simulink library "Library_SII_2018"  (R2018b)
settings: Solver=ode45  StartTime=0.0  StopTime=10.0  RelTol=1e-3  EnableMultiTasking=on
undefined symbols (not defined in the file or in its folder): coder, gcbh, r, simscape
libraries: fl_lib x157, nesl_utility x81, Library_SII2 x44, simulink x17, powerlib x12, mblibv1 x11, Simscape_SII_lib x11, elec_lib x10, Pneumatic_lib x4, $bdroot x2, peRmsMeasurement x1, powerlib_extras x1
(part 6 of 6)

== system Library_SII_2018/Thermique/Paroi (avec convection) ==
  Capacité : fl_lib/Thermal/Thermal Elements/Thermal Mass  mass=masse kg  sp_heat=c J/kg/K  T_specify=on  T_priority=High  T=Ti K  T_nominal_specify=off  T_nominal_unit=K  T_nominal_value=1  Q_specify=off  Q_priority=High  Q=0 J/s  Q_nominal_specify=off  Q_nominal_unit=W  Q_nominal_value=1
  Conduction ext : fl_lib/Thermal/Thermal Elements/Conductive Heat Transfer  area=s m^2  thickness=e/2 cm  th_cond=lambda W/(m*K)  T_specify=off  T_priority=High  T=0 K  T_nominal_specify=off  T_nominal_unit=K  T_nominal_value=1  Q_specify=off  Q_priority=High  Q=0 J/s  Q_nominal_specify=off  Q_nominal_unit=W  Q_nominal_value=1
      settings: SourceProductName=Simscape
  Conduction int : fl_lib/Thermal/Thermal Elements/Conductive Heat Transfer  area=s m^2  thickness=e/2 cm  th_cond=lambda W/(m*K)  T_specify=off  T_priority=High  T=0 K  T_nominal_specify=off  T_nominal_unit=K  T_nominal_value=1  Q_specify=off  Q_priority=High  Q=0 J/s  Q_nominal_specify=off  Q_nominal_unit=W  Q_nominal_value=1
      settings: SourceProductName=Simscape
  Ideal Heat Flow Sensor. : fl_lib/Thermal/Thermal Sensors/Heat Flow Rate Sensor
      settings: SourceProductName=Simscape  SourceProductBaseCode=SS
  Ideal Heat Flow Sensor.1 : fl_lib/Thermal/Thermal Sensors/Heat Flow Rate Sensor
      settings: SourceProductName=Simscape  SourceProductBaseCode=SS
  Ideal Temperature Sensor : fl_lib/Thermal/Thermal Sensors/Temperature Sensor
  PS-Simulink Converter : nesl_utility/PS-Simulink Converter  PhysicalDomain=network_engine_domain  SubClassName=ps_output  LeftPortType=input  RightPortType=output  PseudoPeriodic=off  Frequencies=[]  Unit=degC  AffineConversion=on
  PS2S : nesl_utility/PS-Simulink Converter  PhysicalDomain=network_engine_domain  SubClassName=ps_output  LeftPortType=input  RightPortType=output  PseudoPeriodic=off  Frequencies=[]  Unit=J/s  AffineConversion=off
  PS2S1 : nesl_utility/PS-Simulink Converter  PhysicalDomain=network_engine_domain  SubClassName=ps_output  LeftPortType=input  RightPortType=output  PseudoPeriodic=off  Frequencies=[]  Unit=J/s  AffineConversion=off
  Thermal Reference : fl_lib/Thermal/Thermal Elements/Thermal Reference
  Int : PMIOPort  Side=Left
  Ext : PMIOPort  Port=2  Side=Right
  Ray : PMIOPort  Port=3  Side=Right
  T : Outport
  Fext : Outport  Port=2
  Fint : Outport  Port=3
  wires:
  PS2S1/1 -> Fint/1
  PS2S/1 -> Fext/1
  PS-Simulink Converter/1 -> T/1
  connections:
  Conduction int/RConn1 -- Ideal Heat Flow Sensor.1/LConn1
  Ideal Heat Flow Sensor.1/RConn1 -- PS2S1/LConn1
  Ideal Heat Flow Sensor./RConn1 -- PS2S/LConn1
  Conduction ext/LConn1 -- Ideal Heat Flow Sensor./RConn2
  Conduction ext/RConn1 -- Ext/RConn1
  Int/RConn1 -- Conduction int/LConn1
  Ideal Heat Flow Sensor./LConn1 -- Ideal Temperature Sensor/LConn1 -- Ray/RConn1 -- Ideal Heat Flow Sensor.1/RConn2 -- Capacité/LConn1
  PS-Simulink Converter/LConn1 -- Ideal Temperature Sensor/RConn2
  Thermal Reference/LConn1 -- Ideal Temperature Sensor/RConn1

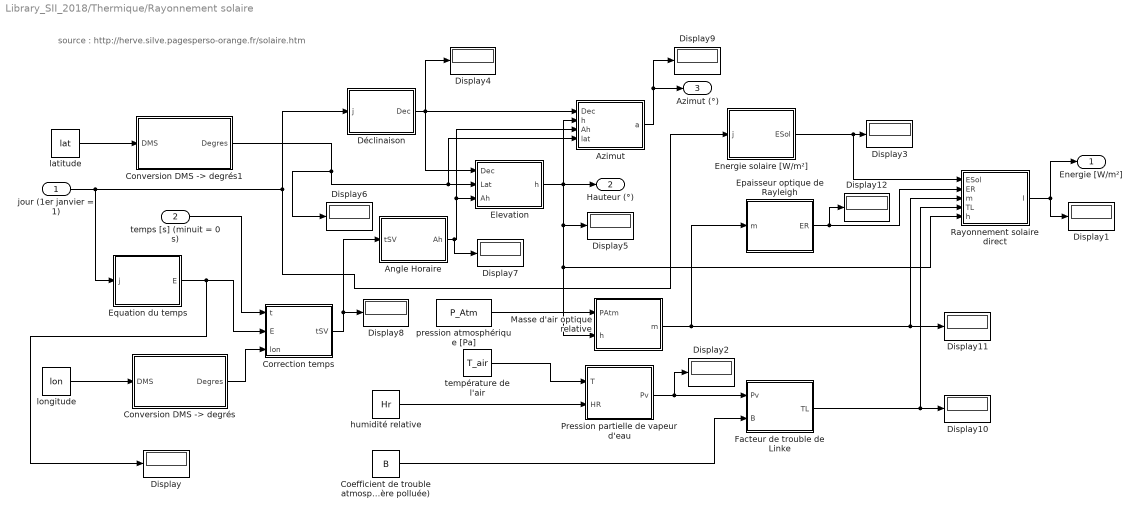
== system Library_SII_2018/Thermique/Rayonnement solaire ==
  note: source : http://herve.silve.pagesperso-orange.fr/solaire.htm
  jour (1er janvier = 1) : Inport
  temps [s] (minuit = 0 s) : Inport  Port=2
  Angle Horaire : MATLAB Function  TreatAsAtomicUnit=on
  Azimut : MATLAB Function  TreatAsAtomicUnit=on
  Coefficient de trouble atmosphérique B = 0,02 pour un lieu situé en montagne B = 0,05 pour un lieu rural B = 0,10 pour un lieu urbain B = 0,20 pour un lieu industriel (atmosphère polluée) : Constant  Value=B
  "Conversion DMS -> degrés" : MATLAB Function  TreatAsAtomicUnit=on
  "Conversion DMS -> degrés1" : MATLAB Function  TreatAsAtomicUnit=on
  Correction temps : MATLAB Function  TreatAsAtomicUnit=on
  Display{,1..12} (13 alike) : Display
  Déclinaison : MATLAB Function  TreatAsAtomicUnit=on
  Elevation : MATLAB Function  TreatAsAtomicUnit=on
  Energie solaire [W/m²] : MATLAB Function  TreatAsAtomicUnit=on
  Epaisseur optique de Rayleigh : MATLAB Function  TreatAsAtomicUnit=on
  Equation du temps : MATLAB Function  TreatAsAtomicUnit=on
  Facteur de trouble de Linke : MATLAB Function  TreatAsAtomicUnit=on
  Masse d'air optique relative : MATLAB Function  TreatAsAtomicUnit=on
  Pression partielle de vapeur d'eau : MATLAB Function  TreatAsAtomicUnit=on
  Rayonnement solaire direct : MATLAB Function  TreatAsAtomicUnit=on
  humidité relative : Constant  Value=Hr
  latitude : Constant  Value=lat
  longitude : Constant  Value=lon
  pression atmosphérique [Pa] : Constant  Value=P_Atm
  température de l'air : Constant  Value=T_air
  Energie [W/m²] : Outport
  Hauteur (°) : Outport  Port=2
  Azimut (°) : Outport  Port=3
  wires:
  Epaisseur optique de Rayleigh/1(ER) -> Display12/1, Rayonnement solaire direct/2(ER)
  Energie solaire [W/m²]/1(ESol) -> Display3/1, Rayonnement solaire direct/1(ESol)
  humidité relative/1 -> Pression partielle de vapeur d'eau/2(HR)
  Rayonnement solaire direct/1(I) -> Energie [W/m²]/1, Display1/1
  température de l'air/1 -> Pression partielle de vapeur d'eau/1(T)
  jour (1er janvier = 1)/1 -> Equation du temps/1(j), Déclinaison/1(j), Energie solaire [W/m²]/1(j)
  Masse d'air optique relative/1(m) -> Display11/1, Rayonnement solaire direct/3(m), Epaisseur optique de Rayleigh/1(m)
  Equation du temps/1(E) -> Display/1, Correction temps/2(E)
  pression atmosphérique [Pa]/1 -> Masse d'air optique relative/1(PAtm)
  Elevation/1(h) -> Azimut/2(h), Masse d'air optique relative/2(h), Rayonnement solaire direct/5(h), Display5/1, Hauteur (°)/1
  Pression partielle de vapeur d'eau/1(Pv) -> Facteur de trouble de Linke/1(Pv), Display2/1
  Facteur de trouble de Linke/1(TL) -> Rayonnement solaire direct/4(TL), Display10/1
  Déclinaison/1(Dec) -> Display4/1, Azimut/1(Dec), Elevation/1(Dec)
  temps [s] (minuit = 0 s)/1 -> Correction temps/1(t)
  Angle Horaire/1(Ah) -> Display7/1, Azimut/3(Ah), Elevation/3(Ah)
  Coefficient de trouble atmosphérique B = 0,02 pour un lieu situé en montagne B = 0,05 pour un lieu rural B = 0,10 pour un lieu urbain B = 0,20 pour un lieu industriel (atmosphère polluée)/1 -> Facteur de trouble de Linke/2(B)
  Correction temps/1(tSV) -> Display8/1, Angle Horaire/1(tSV)
  longitude/1 -> "Conversion DMS -> degrés"/1(DMS)
  "Conversion DMS -> degrés"/1(Degres) -> Correction temps/3(lon)
  "Conversion DMS -> degrés1"/1(Degres) -> Display6/1, Elevation/2(Lat), Azimut/4(lat)
  latitude/1 -> "Conversion DMS -> degrés1"/1(DMS)
  Azimut/1(a) -> Azimut (°)/1, Display9/1

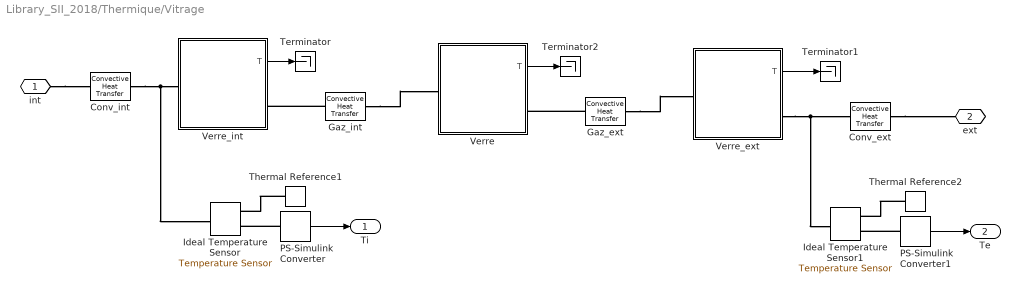
== system Library_SII_2018/Thermique/Vitrage ==
  Conv_ext : fl_lib/Thermal/Thermal Elements/Convective Heat Transfer  area=s m^2  heat_tr_coeff=23 W/(m^2 * K)  T_specify=off  T_priority=High  T=0 K  T_nominal_specify=off  T_nominal_unit=K  T_nominal_value=1  Q_specify=off  Q_priority=High  Q=0 J/s  Q_nominal_specify=off  Q_nominal_unit=W  Q_nominal_value=1
  Conv_int : fl_lib/Thermal/Thermal Elements/Convective Heat Transfer  area=s m^2  heat_tr_coeff=8 W/(m^2 * K)  T_specify=off  T_priority=High  T=0 K  T_nominal_specify=off  T_nominal_unit=K  T_nominal_value=1  Q_specify=off  Q_priority=High  Q=0 J/s  Q_nominal_specify=off  Q_nominal_unit=W  Q_nominal_value=1
  Gaz_ext : fl_lib/Thermal/Thermal Elements/Convective Heat Transfer  area=s m^2  heat_tr_coeff=1e12 W/(m^2 * K)  T_specify=off  T_priority=High  T=0 K  T_nominal_specify=off  T_nominal_unit=K  T_nominal_value=1  Q_specify=off  Q_priority=High  Q=0 J/s  Q_nominal_specify=off  Q_nominal_unit=W  Q_nominal_value=1
  Gaz_int : fl_lib/Thermal/Thermal Elements/Convective Heat Transfer  area=s m^2  heat_tr_coeff=1e12 W/(m^2 * K)  T_specify=off  T_priority=High  T=0 K  T_nominal_specify=off  T_nominal_unit=K  T_nominal_value=1  Q_specify=off  Q_priority=High  Q=0 J/s  Q_nominal_specify=off  Q_nominal_unit=W  Q_nominal_value=1
  Ideal Temperature Sensor : fl_lib/Thermal/Thermal Sensors/Temperature Sensor
  Ideal Temperature Sensor1 : fl_lib/Thermal/Thermal Sensors/Temperature Sensor
  PS-Simulink Converter : nesl_utility/PS-Simulink Converter  PhysicalDomain=network_engine_domain  SubClassName=ps_output  LeftPortType=input  RightPortType=output  PseudoPeriodic=off  Frequencies=[]  Unit=degC  AffineConversion=on
  PS-Simulink Converter1 : nesl_utility/PS-Simulink Converter  PhysicalDomain=network_engine_domain  SubClassName=ps_output  LeftPortType=input  RightPortType=output  PseudoPeriodic=off  Frequencies=[]  Unit=degC  AffineConversion=on
  Terminator : Terminator
  Terminator1 : Terminator
  Terminator2 : Terminator
  Thermal Reference1 : fl_lib/Thermal/Thermal Elements/Thermal Reference
  Thermal Reference2 : fl_lib/Thermal/Thermal Elements/Thermal Reference
  Verre : Subsystem  mask(Paroi){m=Verre, d=off, lambda=1e12, c=720, mv=2530, s=s, e=6, Ti=Ti}
      mask prompts: m "Matériau"; d "Utiliser des valeurs personnalisées"; lambda "Conductivité thermique (W.m<sup>-1</sup>.K<sup>-1</sup>)"; c "Capacité thermique (J.kg<sup>-1</sup>.K<sup>-1</sup>)"; mv "Masse volumique (kg/m<sup>3</sup>)"; s "Surface de la paroi (m<sup>2</sup>)"; e "Epaisseur de la paroi (cm)"; Ti "Température initiale (°C)"
      mask help:
      | Modèle d'une paroi opaque (transmission de la chaleur par conduction).
      |
      | 1) Choisir un matériau
      | ou bien indiquer les caractéristiques thermiques d'un matériau
      | - Conductivité thermique (W.m-1.K-1)
      | - Capacité thermique (J.kg-1.K-1)
      | - Masse volumique (kg/m3)
      |
      | 2) Indiquer les dimensions de la paroi :
      | - Surface (m²)
      | - Epaisseur (cm)
      |
      | 3) Préciser la température initiale (°C)
      |
      | ==> Sortie :
      | T = Température au coeur de la paroi (°C)
      mask init:
      | % Conversion de la température
      | Ti = 273.15+Ti;
      | 
      | % Calcul de la masse
      | masse = mv * s * e / 100;
      | 
      | CaractMateriaux;
      mask Help:
      | Modèle d'une paroi opaque (transmission de la chaleur par conduction).
      | 
      | 1) Choisir un matériau
      | ou bien indiquer les caractéristiques thermiques d'un matériau
      | - Conductivité thermique (W.m<sup>-1</sup>.K<sup>-1</sup>)
      | - Capacité thermique (J.kg<sup>-1</sup>.K<sup>-1</sup>)
      | - Masse volumique (kg/m<sup>3</sup>)
      | 
      | 2) Indiquer les dimensions de la paroi :
      | - Surface (m²)
      | - Epaisseur (cm)
      | 
      | 3) Préciser la température initiale (°C)
      | 
      | ==> Sortie :
      | T = Température au coeur de la paroi (°C)
      | 
      | 
      | Il est possible de trouver les caractéristiques thermiques des principaux
      | matériaux de construction sur le site :
      | <a href="http://www.maison.com/architecture/maison-basse-consommation/quoi-construire-murs-maison-4881/"><tt>www.maison.com</tt></a>
      mask TypeOptions m: Verre
      mask Callback m:
      | CaractMateriaux;
      | dd = get_param(gcb,'d');
      | if strcmp(dd,'off');
      |     mm =  get_param(gcb, 'm');
      |     set_param(gcb, 'lambda',Materiau(mm).Conductivite);
      |     set_param(gcb, 'mv',Materiau(mm).MasseVol);
      |     set_param(gcb, 'c',Materiau(mm).Capacite);
      | end
      mask Callback d:
      | maskStr = get_param(gcb,'MaskValues');
      | dd = get_param(gcb,'d');
      | if strcmp(dd,'on');
      |     set_param(gcb,'MaskEnables',{'on';'on';'on';'on';'on';'on';'on';'on'}),
      | else
      |     set_param(gcb,'MaskEnables',{'on';'on';'off';'off';'off';'on';'on';'on'}),
      | end
      mask Display:
      | image(imread(Materiau(get_param(gcb, 'm')).Image), [0.2, 0, 0.6, 0.85]);
      | port_label('lconn', 1, 'G');
      | port_label('rconn', 1, 'D');
      | port_label('output', 1, 'T');
      | 
      | 
      | text(0.5,0.95, get_param(gcb, 'm'), ...
      |      'HorizontalAlignment','center');
  Verre_ext : Subsystem  mask(Paroi){m=Verre, d=off, lambda=1e12, c=720, mv=2530, s=s, e=3.3, Ti=Ti}
      mask prompts: m "Matériau"; d "Utiliser des valeurs personnalisées"; lambda "Conductivité thermique (W.m<sup>-1</sup>.K<sup>-1</sup>)"; c "Capacité thermique (J.kg<sup>-1</sup>.K<sup>-1</sup>)"; mv "Masse volumique (kg/m<sup>3</sup>)"; s "Surface de la paroi (m<sup>2</sup>)"; e "Epaisseur de la paroi (cm)"; Ti "Température initiale (°C)"
      mask help:
      | Modèle d'une paroi opaque (transmission de la chaleur par conduction).
      |
      | 1) Choisir un matériau
      | ou bien indiquer les caractéristiques thermiques d'un matériau
      | - Conductivité thermique (W.m-1.K-1)
      | - Capacité thermique (J.kg-1.K-1)
      | - Masse volumique (kg/m3)
      |
      | 2) Indiquer les dimensions de la paroi :
      | - Surface (m²)
      | - Epaisseur (cm)
      |
      | 3) Préciser la température initiale (°C)
      |
      | ==> Sortie :
      | T = Température au coeur de la paroi (°C)
      mask init:
      | % Conversion de la température
      | Ti = 273.15+Ti;
      | 
      | % Calcul de la masse
      | masse = mv * s * e / 100;
      | 
      | CaractMateriaux;
      mask Help:
      | Modèle d'une paroi opaque (transmission de la chaleur par conduction).
      | 
      | 1) Choisir un matériau
      | ou bien indiquer les caractéristiques thermiques d'un matériau
      | - Conductivité thermique (W.m<sup>-1</sup>.K<sup>-1</sup>)
      | - Capacité thermique (J.kg<sup>-1</sup>.K<sup>-1</sup>)
      | - Masse volumique (kg/m<sup>3</sup>)
      | 
      | 2) Indiquer les dimensions de la paroi :
      | - Surface (m²)
      | - Epaisseur (cm)
      | 
      | 3) Préciser la température initiale (°C)
      | 
      | ==> Sortie :
      | T = Température au coeur de la paroi (°C)
      | 
      | 
      | Il est possible de trouver les caractéristiques thermiques des principaux
      | matériaux de construction sur le site :
      | <a href="http://www.maison.com/architecture/maison-basse-consommation/quoi-construire-murs-maison-4881/"><tt>www.maison.com</tt></a>
      mask TypeOptions m: Verre
      mask Callback m:
      | CaractMateriaux;
      | dd = get_param(gcb,'d');
      | if strcmp(dd,'off');
      |     mm =  get_param(gcb, 'm');
      |     set_param(gcb, 'lambda',Materiau(mm).Conductivite);
      |     set_param(gcb, 'mv',Materiau(mm).MasseVol);
      |     set_param(gcb, 'c',Materiau(mm).Capacite);
      | end
      mask Callback d:
      | maskStr = get_param(gcb,'MaskValues');
      | dd = get_param(gcb,'d');
      | if strcmp(dd,'on');
      |     set_param(gcb,'MaskEnables',{'on';'on';'on';'on';'on';'on';'on';'on'}),
      | else
      |     set_param(gcb,'MaskEnables',{'on';'on';'off';'off';'off';'on';'on';'on'}),
      | end
      mask Display:
      | image(imread(Materiau(get_param(gcb, 'm')).Image), [0.2, 0, 0.6, 0.85]);
      | port_label('lconn', 1, 'G');
      | port_label('rconn', 1, 'D');
      | port_label('output', 1, 'T');
      | 
      | 
      | text(0.5,0.95, get_param(gcb, 'm'), ...
      |      'HorizontalAlignment','center');
  Verre_int : Subsystem  mask(Paroi){m=Verre, d=off, lambda=1.2, c=720, mv=2530, s=s, e=4, Ti=Ti}
      mask prompts: m "Matériau"; d "Utiliser des valeurs personnalisées"; lambda "Conductivité thermique (W.m<sup>-1</sup>.K<sup>-1</sup>)"; c "Capacité thermique (J.kg<sup>-1</sup>.K<sup>-1</sup>)"; mv "Masse volumique (kg/m<sup>3</sup>)"; s "Surface de la paroi (m<sup>2</sup>)"; e "Epaisseur de la paroi (cm)"; Ti "Température initiale (°C)"
      mask help:
      | Modèle d'une paroi opaque (transmission de la chaleur par conduction).
      |
      | 1) Choisir un matériau
      | ou bien indiquer les caractéristiques thermiques d'un matériau
      | - Conductivité thermique (W.m-1.K-1)
      | - Capacité thermique (J.kg-1.K-1)
      | - Masse volumique (kg/m3)
      |
      | 2) Indiquer les dimensions de la paroi :
      | - Surface (m²)
      | - Epaisseur (cm)
      |
      | 3) Préciser la température initiale (°C)
      |
      | ==> Sortie :
      | T = Température au coeur de la paroi (°C)
      mask init:
      | % Conversion de la température
      | Ti = 273.15+Ti;
      | 
      | % Calcul de la masse
      | masse = mv * s * e / 100;
      | 
      | CaractMateriaux;
      mask Help:
      | Modèle d'une paroi opaque (transmission de la chaleur par conduction).
      | 
      | 1) Choisir un matériau
      | ou bien indiquer les caractéristiques thermiques d'un matériau
      | - Conductivité thermique (W.m<sup>-1</sup>.K<sup>-1</sup>)
      | - Capacité thermique (J.kg<sup>-1</sup>.K<sup>-1</sup>)
      | - Masse volumique (kg/m<sup>3</sup>)
      | 
      | 2) Indiquer les dimensions de la paroi :
      | - Surface (m²)
      | - Epaisseur (cm)
      | 
      | 3) Préciser la température initiale (°C)
      | 
      | ==> Sortie :
      | T = Température au coeur de la paroi (°C)
      | 
      | 
      | Il est possible de trouver les caractéristiques thermiques des principaux
      | matériaux de construction sur le site :
      | <a href="http://www.maison.com/architecture/maison-basse-consommation/quoi-construire-murs-maison-4881/"><tt>www.maison.com</tt></a>
      mask TypeOptions m: Verre
      mask Callback m:
      | CaractMateriaux;
      | dd = get_param(gcb,'d');
      | if strcmp(dd,'off');
      |     mm =  get_param(gcb, 'm');
      |     set_param(gcb, 'lambda',Materiau(mm).Conductivite);
      |     set_param(gcb, 'mv',Materiau(mm).MasseVol);
      |     set_param(gcb, 'c',Materiau(mm).Capacite);
      | end
      mask Callback d:
      | maskStr = get_param(gcb,'MaskValues');
      | dd = get_param(gcb,'d');
      | if strcmp(dd,'on');
      |     set_param(gcb,'MaskEnables',{'on';'on';'on';'on';'on';'on';'on';'on'}),
      | else
      |     set_param(gcb,'MaskEnables',{'on';'on';'off';'off';'off';'on';'on';'on'}),
      | end
      mask Display:
      | image(imread(Materiau(get_param(gcb, 'm')).Image), [0.2, 0, 0.6, 0.85]);
      | port_label('lconn', 1, 'G');
      | port_label('rconn', 1, 'D');
      | port_label('output', 1, 'T');
      | 
      | 
      | text(0.5,0.95, get_param(gcb, 'm'), ...
      |      'HorizontalAlignment','center');
  int : PMIOPort  Side=Left
  ext : PMIOPort  Port=2  Side=Right
  Ti : Outport
  Te : Outport  Port=2
  wires:
  Verre_int/1(T) -> Terminator/1
  Verre_ext/1(T) -> Terminator1/1
  Verre/1(T) -> Terminator2/1
  PS-Simulink Converter/1 -> Ti/1
  PS-Simulink Converter1/1 -> Te/1
  connections:
  Gaz_int/LConn1 -- Verre_int/RConn1
  int/RConn1 -- Conv_int/LConn1
  Conv_int/RConn1 -- Verre_int/LConn1 -- Ideal Temperature Sensor/LConn1
  Verre_ext/RConn1 -- Conv_ext/LConn1 -- Ideal Temperature Sensor1/LConn1
  Conv_ext/RConn1 -- ext/RConn1
  Gaz_ext/LConn1 -- Verre/RConn1
  PS-Simulink Converter/LConn1 -- Ideal Temperature Sensor/RConn2
  Thermal Reference1/LConn1 -- Ideal Temperature Sensor/RConn1
  PS-Simulink Converter1/LConn1 -- Ideal Temperature Sensor1/RConn2
  Thermal Reference2/LConn1 -- Ideal Temperature Sensor1/RConn1
  Gaz_ext/RConn1 -- Verre_ext/LConn1
  Gaz_int/RConn1 -- Verre/LConn1

== system Library_SII_2018/Electromécanique/Moteur CC (SPS-SM)/Actionneur en vitesse ==
  signal : Inport
  Derivative : Derivative
  Integrator : Integrator
  Joint Actuator : mblibv1/Sensors &  Actuators/Joint Actuator  UpdateFromCAD=off  PhysicalDomain=Mechanical  PortType=blob  ActuationStyle=Motion  AngleUnits=rad  ArcVelocityUnits=rad/s  ArcAccelerationUnits=rad/s^2  CoordPositionUnits=m  VelocityUnits=m/s  AccelerationUnits=m/s^2  ForceUnits=N  TorqueUnits=N*m  ActiveIO=off  Width=3  DialogClass=MechanicalActuatorBlock  Primitive=R1  ReferenceFrame=Absolute (World)
      settings: SourceProductName=Simscape Multibody  SourceProductBaseCode=MS
  Mux1 : Mux  Inputs=3
  liaison : PMIOPort  Side=Right
  wires:
  Derivative/1 -> Mux1/3
  Integrator/1 -> Mux1/1
  Mux1/1 -> Joint Actuator/1
  signal/1 -> Mux1/2, Derivative/1, Integrator/1
  connections:
  liaison/RConn1 -- Joint Actuator/RConn1

== system Library_SII_2018/Electronique/Cellule Photovoltaique SPS/Courant de saturation diode ==
  Tj : Inport
  Vt : Inport  Port=2
  Fcn : Fcn  Expr=I0d*((u(1)+Kel)/(Tjref+Kel))^(TXI/N)*exp(EG*((u(1)+Kel)/(Tjref+Kel)-1)/(N*u(2)))
  Mux : Mux  Inputs=2
  Id0 : Outport
  wires:
  Fcn/1 -> Id0/1
  Mux/1 -> Fcn/1
  Tj/1 -> Mux/1
  Vt/1 -> Mux/2

== system Library_SII_2018/Electronique/Cellule Photovoltaique SPS/Courant diode ==
  Vd : Inport
  I0d : Inport  Port=2
  Vt : Inport  Port=3
  Fcn : Fcn  Expr=u(2)*(exp(u(1)/u(3)/N) - 1)
  Mux : Mux  Inputs=3
  Id : Outport
  wires:
  Fcn/1 -> Id/1
  Mux/1 -> Fcn/1
  Vd/1 -> Mux/1
  I0d/1 -> Mux/2
  Vt/1 -> Mux/3

== system Library_SII_2018/Electronique/Cellule Photovoltaique SPS/Courant gégéré par l'éclairement ==
  Tj : Inport
  Ir : Inport  Port=2
  Fcn : Fcn  Expr=I0*u(2)/Eref*(1+alpha*(u(1)-Tjref))
  Mux : Mux  Inputs=2
  Iph : Outport
  wires:
  Ir/1 -> Mux/2
  Fcn/1 -> Iph/1
  Tj/1 -> Mux/1
  Mux/1 -> Fcn/1

== system Library_SII_2018/Electronique/Cellule Photovoltaique SPS/Estimation température cellule ==
  note: Estimation de la température de la cellule
      | Ta en °C
      | Es en W/m²
      | Tj en °C
  noct : Inport
  Ta : Inport  Port=2
  Ir : Inport  Port=3
  Fcn : Fcn  Expr=u(2)+u(3)*((u(1)-20)/800)
  Mux : Mux  Inputs=3
  Tj : Outport
  wires:
  Ir/1 -> Mux/3
  Ta/1 -> Mux/2
  Fcn/1 -> Tj/1
  noct/1 -> Mux/1
  Mux/1 -> Fcn/1

== system Library_SII_2018/Electronique/Cellule Photovoltaique SPS/Tension thermique ==
  Tj (°C) : Inport
  Fcn : Fcn  Expr=k*(u+Kel)/q
  Vt (V) : Outport
  wires:
  Fcn/1 -> Vt (V)/1
  Tj (°C)/1 -> Fcn/1

== system Library_SII_2018/Electronique/Diode/Courant de saturation diode ==
  Tj : Inport
  Fcn : Fcn  Expr=I0d
  Id0 : Outport
  wires:
  Fcn/1 -> Id0/1
  Tj/1 -> Fcn/1

== system Library_SII_2018/Electronique/Diode/Courant diode ==
  Vd : Inport
  I0d : Inport  Port=2
  Vt : Inport  Port=3
  Fcn : Fcn  Expr=u(2)*(exp(u(1)/u(3)/N) - 1)
  Mux : Mux  Inputs=3
  Id : Outport
  wires:
  Fcn/1 -> Id/1
  Mux/1 -> Fcn/1
  Vd/1 -> Mux/1
  I0d/1 -> Mux/2
  Vt/1 -> Mux/3

== system Library_SII_2018/Electronique/Diode/Tension thermique ==
  Tj (°C) : Inport
  Fcn : Fcn  Expr=k*(u+Kel)/q
  Vt : Outport
  wires:
  Fcn/1 -> Vt/1
  Tj (°C)/1 -> Fcn/1

== system Library_SII_2018/Mécanique/Engrenage droit SS/Capteur de puissance mécanique de rotation ==
  Ideal Rotational Motion Sensor : fl_lib/Mechanical/Mechanical Sensors/Ideal Rotational Motion Sensor  offset=0 rad
  Ideal Torque Sensor : fl_lib/Mechanical/Mechanical Sensors/Ideal Torque Sensor
  PS-Simulink Converter : nesl_utility/PS-Simulink Converter  PhysicalDomain=network_engine_domain  SubClassName=ps_output  LeftPortType=input  RightPortType=output  PseudoPeriodic=off  Frequencies=[]  Unit=1  AffineConversion=off
  PS-Simulink Converter1 : nesl_utility/PS-Simulink Converter  PhysicalDomain=network_engine_domain  SubClassName=ps_output  LeftPortType=input  RightPortType=output  PseudoPeriodic=off  Frequencies=[]  Unit=1  AffineConversion=off
  Product : Product  RndMeth=Zero
  Ref : PMIOPort  Tag=PMCPort  Side=Left
  E : PMIOPort  Port=2  Side=Left
  S : PMIOPort  Tag=PMCPort  Port=3  Side=Right
  P : Outport
  C : Outport  Port=2
  W : Outport  Port=3
  wires:
  PS-Simulink Converter/1 -> C/1, Product/1
  PS-Simulink Converter1/1 -> W/1, Product/2
  Product/1 -> P/1
  connections:
  Ideal Torque Sensor/LConn1 -- E/RConn1
  Ideal Torque Sensor/RConn1 -- S/RConn1 -- Ideal Rotational Motion Sensor/RConn1
  Ideal Rotational Motion Sensor/LConn1 -- Ref/RConn1
  Ideal Rotational Motion Sensor/RConn2 -- PS-Simulink Converter1/LConn1
  Ideal Torque Sensor/RConn2 -- PS-Simulink Converter/LConn1

== system Library_SII_2018/Mécanique/Roue - Vis sans fin SS/Capteur de puissance mécanique de rotation ==
  Ideal Rotational Motion Sensor : fl_lib/Mechanical/Mechanical Sensors/Ideal Rotational Motion Sensor  offset=0 rad
  Ideal Torque Sensor : fl_lib/Mechanical/Mechanical Sensors/Ideal Torque Sensor
  PS-Simulink Converter : nesl_utility/PS-Simulink Converter  PhysicalDomain=network_engine_domain  SubClassName=ps_output  LeftPortType=input  RightPortType=output  PseudoPeriodic=off  Frequencies=[]  Unit=1  AffineConversion=off
  PS-Simulink Converter1 : nesl_utility/PS-Simulink Converter  PhysicalDomain=network_engine_domain  SubClassName=ps_output  LeftPortType=input  RightPortType=output  PseudoPeriodic=off  Frequencies=[]  Unit=1  AffineConversion=off
  Product : Product  RndMeth=Zero
  Ref : PMIOPort  Tag=PMCPort  Side=Left
  E : PMIOPort  Port=2  Side=Left
  S : PMIOPort  Tag=PMCPort  Port=3  Side=Right
  P : Outport
  C : Outport  Port=2
  W : Outport  Port=3
  wires:
  PS-Simulink Converter/1 -> C/1, Product/1
  PS-Simulink Converter1/1 -> W/1, Product/2
  Product/1 -> P/1
  connections:
  Ideal Torque Sensor/LConn1 -- E/RConn1
  Ideal Torque Sensor/RConn1 -- S/RConn1 -- Ideal Rotational Motion Sensor/RConn1
  Ideal Rotational Motion Sensor/LConn1 -- Ref/RConn1
  Ideal Rotational Motion Sensor/RConn2 -- PS-Simulink Converter1/LConn1
  Ideal Torque Sensor/RConn2 -- PS-Simulink Converter/LConn1

== system Library_SII_2018/Thermique/Vitrage/Verre ==
  Conductive_ext : fl_lib/Thermal/Thermal Elements/Conductive Heat Transfer  area=s m^2  thickness=e/2 mm  th_cond=lambda W/(m*K)  T_specify=off  T_priority=High  T=0 K  T_nominal_specify=off  T_nominal_unit=K  T_nominal_value=1  Q_specify=off  Q_priority=High  Q=0 J/s  Q_nominal_specify=off  Q_nominal_unit=W  Q_nominal_value=1
      settings: SourceProductName=Simscape
  Conductive_int : fl_lib/Thermal/Thermal Elements/Conductive Heat Transfer  area=s m^2  thickness=e/2 mm  th_cond=lambda W/(m*K)  T_specify=off  T_priority=High  T=0 K  T_nominal_specify=off  T_nominal_unit=K  T_nominal_value=1  Q_specify=off  Q_priority=High  Q=0 J/s  Q_nominal_specify=off  Q_nominal_unit=W  Q_nominal_value=1
      settings: SourceProductName=Simscape
  Ideal Temperature Sensor : fl_lib/Thermal/Thermal Sensors/Temperature Sensor
  Inertie : fl_lib/Thermal/Thermal Elements/Thermal Mass  mass=masse kg  sp_heat=c J/kg/K  T_specify=on  T_priority=High  T=Ti K  T_nominal_specify=off  T_nominal_unit=K  T_nominal_value=1  Q_specify=off  Q_priority=High  Q=0 J/s  Q_nominal_specify=off  Q_nominal_unit=W  Q_nominal_value=1
  PS-Simulink Converter : nesl_utility/PS-Simulink Converter  PhysicalDomain=network_engine_domain  SubClassName=ps_output  LeftPortType=input  RightPortType=output  PseudoPeriodic=off  Frequencies=[]  Unit=degC  AffineConversion=on
  Thermal Reference1 : fl_lib/Thermal/Thermal Elements/Thermal Reference
  L : PMIOPort  Side=Left
  R : PMIOPort  Port=2  Side=Right
  T : Outport
  wires:
  PS-Simulink Converter/1 -> T/1
  connections:
  Conductive_ext/LConn1 -- Conductive_int/RConn1 -- Inertie/LConn1 -- Ideal Temperature Sensor/LConn1
  L/RConn1 -- Conductive_int/LConn1
  R/RConn1 -- Conductive_ext/RConn1
  PS-Simulink Converter/LConn1 -- Ideal Temperature Sensor/RConn2
  Thermal Reference1/LConn1 -- Ideal Temperature Sensor/RConn1

== system Library_SII_2018/Thermique/Vitrage/Verre_ext ==
  Conductive_ext : fl_lib/Thermal/Thermal Elements/Conductive Heat Transfer  area=s m^2  thickness=e/2 mm  th_cond=lambda W/(m*K)  T_specify=off  T_priority=High  T=0 K  T_nominal_specify=off  T_nominal_unit=K  T_nominal_value=1  Q_specify=off  Q_priority=High  Q=0 J/s  Q_nominal_specify=off  Q_nominal_unit=W  Q_nominal_value=1
      settings: SourceProductName=Simscape
  Conductive_int : fl_lib/Thermal/Thermal Elements/Conductive Heat Transfer  area=s m^2  thickness=e/2 mm  th_cond=lambda W/(m*K)  T_specify=off  T_priority=High  T=0 K  T_nominal_specify=off  T_nominal_unit=K  T_nominal_value=1  Q_specify=off  Q_priority=High  Q=0 J/s  Q_nominal_specify=off  Q_nominal_unit=W  Q_nominal_value=1
      settings: SourceProductName=Simscape
  Ideal Temperature Sensor : fl_lib/Thermal/Thermal Sensors/Temperature Sensor
  Inertie : fl_lib/Thermal/Thermal Elements/Thermal Mass  mass=masse kg  sp_heat=c J/kg/K  T_specify=on  T_priority=High  T=Ti K  T_nominal_specify=off  T_nominal_unit=K  T_nominal_value=1  Q_specify=off  Q_priority=High  Q=0 J/s  Q_nominal_specify=off  Q_nominal_unit=W  Q_nominal_value=1
  PS-Simulink Converter : nesl_utility/PS-Simulink Converter  PhysicalDomain=network_engine_domain  SubClassName=ps_output  LeftPortType=input  RightPortType=output  PseudoPeriodic=off  Frequencies=[]  Unit=degC  AffineConversion=on
  Thermal Reference1 : fl_lib/Thermal/Thermal Elements/Thermal Reference
  L : PMIOPort  Side=Left
  R : PMIOPort  Port=2  Side=Right
  T : Outport
  wires:
  PS-Simulink Converter/1 -> T/1
  connections:
  Thermal Reference1/LConn1 -- Ideal Temperature Sensor/RConn1
  PS-Simulink Converter/LConn1 -- Ideal Temperature Sensor/RConn2
  R/RConn1 -- Conductive_ext/RConn1
  L/RConn1 -- Conductive_int/LConn1
  Ideal Temperature Sensor/LConn1 -- Inertie/LConn1 -- Conductive_int/RConn1 -- Conductive_ext/LConn1

== system Library_SII_2018/Thermique/Vitrage/Verre_int ==
  Conductive_ext : fl_lib/Thermal/Thermal Elements/Conductive Heat Transfer  area=s m^2  thickness=e/2 mm  th_cond=lambda W/(m*K)  T_specify=off  T_priority=High  T=0 K  T_nominal_specify=off  T_nominal_unit=K  T_nominal_value=1  Q_specify=off  Q_priority=High  Q=0 J/s  Q_nominal_specify=off  Q_nominal_unit=W  Q_nominal_value=1
      settings: SourceProductName=Simscape
  Conductive_int : fl_lib/Thermal/Thermal Elements/Conductive Heat Transfer  area=s m^2  thickness=e/2 cm  th_cond=lambda W/(m*K)  T_specify=off  T_priority=High  T=0 K  T_nominal_specify=off  T_nominal_unit=K  T_nominal_value=1  Q_specify=off  Q_priority=High  Q=0 J/s  Q_nominal_specify=off  Q_nominal_unit=W  Q_nominal_value=1
      settings: SourceProductName=Simscape
  Ideal Temperature Sensor : fl_lib/Thermal/Thermal Sensors/Temperature Sensor
  Inertie : fl_lib/Thermal/Thermal Elements/Thermal Mass  mass=masse kg  sp_heat=c J/kg/K  T_specify=on  T_priority=High  T=Ti K  T_nominal_specify=off  T_nominal_unit=K  T_nominal_value=1  Q_specify=off  Q_priority=High  Q=0 J/s  Q_nominal_specify=off  Q_nominal_unit=W  Q_nominal_value=1
  PS-Simulink Converter : nesl_utility/PS-Simulink Converter  PhysicalDomain=network_engine_domain  SubClassName=ps_output  LeftPortType=input  RightPortType=output  PseudoPeriodic=off  Frequencies=[]  Unit=degC  AffineConversion=on
  Thermal Reference1 : fl_lib/Thermal/Thermal Elements/Thermal Reference
  L : PMIOPort  Side=Left
  R : PMIOPort  Port=2  Side=Right
  T : Outport
  wires:
  PS-Simulink Converter/1 -> T/1
  connections:
  Thermal Reference1/LConn1 -- Ideal Temperature Sensor/RConn1
  PS-Simulink Converter/LConn1 -- Ideal Temperature Sensor/RConn2
  R/RConn1 -- Conductive_ext/RConn1
  L/RConn1 -- Conductive_int/LConn1
  Ideal Temperature Sensor/LConn1 -- Inertie/LConn1 -- Conductive_int/RConn1 -- Conductive_ext/LConn1

== matlab function Library_SII_2018/Signaux/Contrôle de régime/MATLAB Function ==
  data: t input; t_1 input; x input; xc output; al input; vl input; x_1 input; v_1 input
function xc = fcn(t, t_1, x, al, vl, x_1, v_1)
%#codegen
if t_1>0
    p = 5;
    v = v_1;
    
%     if v>0 && x_1 >= x
%         xc = x;
%         return
%     end
    
    if v > 0
%         xl = v^2/(2*al)+x_1;
        ac = -v^2/(x-x_1)/2;
    elseif v < 0
%         xl = -v^2/(2*al)+x_1;
        ac = -v^2/(x-x_1)/2;
    else
        ac = 0;
    end

    if v>0 && ac <= -al
        acc = -al;
        v0 = v;
    elseif v<0 && ac >= al
        acc = al;
        v0 = v;
%     elseif v>0 && ac <= -al*(1-1/p)
%         acc = -al
%         v0 = v;
%     elseif v<0 && ac >= al*(1-1/p)
%         acc = ac*(1+1/p);
%         v0 = v;
    else
        if v >= vl
            acc = 0;
            v0 = vl;
        elseif v <= -vl
            acc = 0;
            v0 = -vl;
        else
            
            if x_1 < x
                acc = al;
                v0 = v;
            elseif x_1 > x
                acc = -al;
                v0 = v;
            else
                acc = 0;
                v0 = 0;
            end
        end
    end
    
    xc = acc*(t-t_1)^2 + v0*(t-t_1) + x_1;
    
    v = (xc-x_1)/(t-t_1);
    if abs(v) > vl
        xc = sign(v)*vl*(t-t_1)+x_1;
    end
    
    if (xc-x) * (x_1-x) <= 0
        xc = x;
    end
    
else
    xc = 0;
end

== matlab function Library_SII_2018/Signaux/Frequence-Metre/MATLAB Function ==
  data: x input; F output; fs input; Pmax output; spec input; plage input
function [F, Pmax] = Frequence( x, fs , spec, plage)
%UNTITLED Summary of this function goes here
%   Detailed explanation goes here

m = length(x);          % Window length
n = pow2(nextpow2(m));  % Transform length
y = fft(x,n)/m;           % DFT

f = fs/2*linspace(0,1,n/2+1);


power = 2*abs(y(1:n/2+1));
np = length(power);

[Pmax, I] = max(power(2:np));
F = f(I+1);

coder.extrinsic('plot');
if spec == 1;
    i_d = find(f>plage(1));
    i_f = find(f>plage(2));
    if isempty(i_d) | plage(1) == -1;
        i_d = 1;
    else 
        i_d = i_d(1);
    end
    if isempty(i_f) | plage(2) == -1;
        i_f = length(f);
    else
        i_f = i_f(1);
    end
    f = f(i_d:i_f);
    power = power(i_d:i_f);
    plot(f,power);
end

end

== stateflow chart Library_SII_2018/Signaux/Codeur incrémental/Chart ==
  (default) -> (junction 13) : {y=1;}
  data: y output
  events: hold input RISING_EDGE_EVENT

== matlab function Library_SII_2018/Thermique/Incidence surface/Coefficient d'incidence ==
  data: i input; CI output; o input; h input; a input
function CI = fcn(i, o, h, a)
%#codegen
CI = sind(i) * cosd(h) * cosd(o - 180+a) + cosd(i) * sind(h);
if CI < 0
    % Surface à l'ombre
    CI = 0;
end;

== stateflow chart Library_SII_2018/Signaux/Codeur incrémental/bascule A ==
  state haut
    en:
    s=0;
    t=0;
  state bas
    en:
    s = 1;
    t=1;
  bas -> haut : top
  haut -> bas : top
  (default) -> bas : top
  data: s output; t output
  events: top input RISING_EDGE_EVENT

== stateflow chart Library_SII_2018/Signaux/Codeur incrémental/bascule B ==
  state haut
    en:
    s=0;
    t=0;
  state bas
    en:
    s = 1;
    t=1;
  bas -> haut : top
  haut -> bas : top
  (default) -> bas : top
  data: s output; t output
  events: top input RISING_EDGE_EVENT

== stateflow chart Library_SII_2018/Signaux/bascule ==
  state haut
    en:s=0;
  state bas
    en:s = 1;
  haut -> bas : top
  bas -> haut : top
  (default) -> bas : top
  data: s output
  events: top input RISING_EDGE_EVENT

== stateflow chart Library_SII_2018/Signaux/bascule 2 sorties ==
  state haut
    en:
    s=0;
    t=0;
  state bas
    en:
    s = 1;
    t=1;
  bas -> haut : top
  haut -> bas : top
  (default) -> bas : top
  data: s output; t output
  events: top input RISING_EDGE_EVENT

== stateflow chart Library_SII_2018/Electromécanique/Décodeur pour codeur incrémental/Décodeur position - vitesse accélération - fréquence ==
  state top
    en:
    dt = t-t_;
    if A~=B
    p = p - k;
    else
    p = p + k;
    end
    if dt>0
    dp = p-p_;
    v = dp/dt;
    a = (v-v_)/dt;
    else
    v = 0;
    a = 0;
    end
    p_ = p;
    v_ = v;
    t_ = t;
    % Fréquence de filtrage
    f = 1/(5*dt);
  top -> top : fA
  (default) -> top : {p=0;v=0;a=0;v_=0;t_=0;p_=0;}
  data: A input; B input; p output; v output; a output; v_ local; p_ local; t_ local; k input; t input; dt local; dp local; f output
  events: fA input EITHER_EDGE_EVENT

== matlab function Library_SII_2018/Mécanique/Corde/Calcul de la raideur ==
  data: E input; k output; S input; L input
function k = fcn(E, S, L)
%#codegen

k = S*E/L;

== matlab function Library_SII_2018/Electromécanique/Décodeur pour codeur incrémental/MATLAB Function ==
  data: u input; y output; inv input
function y = fcn(u, inv)
%#codegen
if inv
    y = -u;
else
    y = u;
end

== matlab function Library_SII_2018/Electromécanique/Pont en H/Commande du pont en H ==
  data: mode input; a output; b output; c output; d output
function [a, b, c, d]= fcn(mode)
% mode de fonctionnement
% +1 : avant
% -1 : arrière
% 0 : libre
% 2 : freinage

if mode == 1
    a = 1;
    d = 1;
    b = 0;
    c = 0;
elseif mode == -1
    a = 0;
    d = 0;
    b = 1;
    c = 1;
elseif mode == 0
    a = 0;
    d = 0;
    b = 0;
    c = 0;
else
    a = 0;
    d = 1;
    b = 0;
    c = 1;
end

== matlab function Library_SII_2018/Electromécanique/Servomoteur modèle de connaissance/Commande du pont en H ==
  data: da input; a output; b output; c output; d output; res input
function [a, b, c, d]= fcn(da, res)
%#codegen
sens = sign(da);
ecart = abs(da);
if ecart > res
    if sens > 0
        a = 1;
        d = 1;
        b = 0;
        c = 0;
    else
        a = 0;
        d = 0;
        b = 1;
        c = 1;
    end
else
    a = 0;
    d = 1;
    b = 0;
    c = 1;
end

== stateflow chart Library_SII_2018/Electromécanique/Servomoteur modèle de connaissance/Echantillonage ==
  state top
    en: s=e;
  (default) -> top
  top -> top : after(t, sec)
  data: t input; e input; s output

== matlab function Library_SII_2018/Thermique/Rayonnement solaire/Angle Horaire ==
  data: tSV input; Ah output
function Ah = fcn(tSV)
%#codegen
Ah = 360 * (tSV - 12) / 24 ;

== matlab function Library_SII_2018/Thermique/Rayonnement solaire/Azimut ==
  data: Dec input; h input; Ah input; a output; lat input
function a = fcn(Dec, h, Ah, lat)
%#codegen
a = acosd((sind(Dec)-sind(lat)*sind(h))/(cosd(lat)*cosd(h)));
sinazimut = (cosd(Dec)*sind(Ah))/cosd(h);
if sinazimut < 0
    a = 360-a;
end;

== stateflow chart Library_SII_2018/Automatisme/Vérin/Vérin A ==
  state Aller
    entry:
    s = 0;
    r = 0;
  state Sorti
    entry:
    s = 1;
  state Rentre
    entry:
    r = 1;
  state Retour
    entry:
    s = 0;
    r = 0;
  Aller -> Aller [order 2] : [after(T/N, sec)]{x=x+1;}
  Rentre -> Aller : [S]
  Aller -> Sorti [order 1] : [x==N]
  (default) -> Rentre : {x=0;}
  Sorti -> Retour : [~S]
  Retour -> Rentre [order 1] : [x==0]
  Retour -> Retour [order 2] : [after(T/N, sec)]{x=x-1;}
  data: r output; s output; S input; T input double; x output; N input

== matlab function Library_SII_2018/Thermique/Rayonnement solaire/Conversion DMS -> degrés ==
  data: DMS input; Degres output
function Degres = fcn(DMS)
%#codegen
if DMS(1) >= 0
    Degres = DMS(1) + DMS(2)/60 + DMS(3)/3600;
else
    Degres = DMS(1) - DMS(2)/60 - DMS(3)/3600;
end;

== matlab function Library_SII_2018/Thermique/Rayonnement solaire/Conversion DMS -> degrés1 ==
  data: DMS input; Degres output
function Degres = fcn(DMS)
%#codegen
if DMS(1) >= 0
    Degres = DMS(1) + DMS(2)/60 + DMS(3)/3600;
else
    Degres = DMS(1) - DMS(2)/60 - DMS(3)/3600;
end;

== matlab function Library_SII_2018/Thermique/Rayonnement solaire/Correction temps ==
  data: t input; E input; lon input; tSV output
function tSV = fcn(t, E, lon)
%#codegen
tSV = t/3600 - 1 - E/60 - 4*lon/60;

== matlab function Library_SII_2018/Thermique/Rayonnement solaire/Déclinaison ==
  data: j input; Dec output
function Dec = fcn(j)
%#codegen
va = 360/360.25;
Dec = asind(0.3978 * sind(va * (j - (81 - 2 * sind(va * (j - 2))))));

== matlab function Library_SII_2018/Thermique/Rayonnement solaire/Elevation ==
  data: Dec input; Lat input; Ah input; h output
function h = fcn(Dec, Lat, Ah)
%#codegen
h = asind(sind(Lat) * sind(Dec) + cosd(Lat) * cosd(Dec) * cosd(Ah));
if h < 0
    h = 0;
end;

== matlab function Library_SII_2018/Thermique/Rayonnement solaire/Energie solaire [W//m²] ==
  data: j input; ESol output
function ESol = fcn(j)
%#codegen
ESol = 1367 * (1 + 0.0334 * cosd(360 * (j - 2.7206) / 365.25));

== matlab function Library_SII_2018/Thermique/Rayonnement solaire/Epaisseur optique de Rayleigh ==
  data: m input; ER output
function ER = fcn(m)
%#codegen
ER = 1 / (0.9 * m + 9.4);

== matlab function Library_SII_2018/Thermique/Rayonnement solaire/Equation du temps ==
  data: j input; E output
function E = fcn(j)
%#codegen
C = (1.9148 * sind(357.5291 + 0.98560028 * j) + 0.02 * sind(2 * (357.5291 + 0.98560028 * j)) + 0.0003 * sind(3 * (357.5291+0.98560028 * j))) * 4;
O = (-2.468 * sind(2 * (280.4665 + 0.98564736 * j)) + 0.053 * sind(4 * (280.4665 + 0.98564736 * j)) - 0.0014 * sind(6 * (280.4665 + 0.98564736 * j))) * 4;
E = C + O;

== matlab function Library_SII_2018/Thermique/Rayonnement solaire/Facteur de trouble de Linke ==
  data: Pv input; B input; TL output
function TL = fcn(Pv, B)
%#codegen
TL = 2.4 + 14.6 * B + 0.4 * (1 + 2 * B) * log(Pv);

== matlab function Library_SII_2018/Thermique/Rayonnement solaire/Masse d'air optique relative ==
  data: PAtm input; m output; h input
function m = fcn(PAtm, h)
%#codegen
m = PAtm / (101325 * sind(h) + 15198.75 * (3.885 + h)^-1.253);

== matlab function Library_SII_2018/Thermique/Rayonnement solaire/Pression partielle de vapeur d'eau ==
  data: T input; Pv output; HR input
function Pv = fcn(T, HR)
%#codegen
Pvs = 2.165 * (1.098 + T / 100)^8.02;
Pv = Pvs * HR;

== matlab function Library_SII_2018/Thermique/Rayonnement solaire/Rayonnement solaire direct ==
  data: ESol input; ER input; I output; m input; TL input; h input
function I = fcn(ESol, ER, m, TL, h)
%#codegen
if h == 0
    I = 0;
else
    I = ESol * exp(-ER * m * TL);
end;

== matlab function Library_SII_2018/Signaux/Tracé XY point à point ==
  data: x input; y input; xmin parameter; xmax parameter; ymin parameter; ymax parameter
function fcn(x, y, xmin, xmax, ymin, ymax)
coder.extrinsic('plot')
coder.extrinsic('gcb')
coder.extrinsic('get_param')

% Get the mask object
%mo = get_param(gcb,'MaskObject');
%titre = mo.Parameters(1).Value;%
%p = Simulink.Mask.get(gcb);
%titre = p.getParameter('titre');


titre = get_param(gcb, 'titre');
style = get_param(gcb, 'style');
%figure(f);
fh = findobj( 'Type', 'Figure', 'Name', titre);
if ~isempty(fh)
    set(0,'CurrentFigure',fh(1));
    %figure(fh(1));
end

plot(x,y,style)%,'-o','Markersize',6,'MarkerFaceColor','g');
